simulink model "aocs"  (R2026a)
settings: Solver=VariableStepAuto  StopTime=500
values from neighbouring files (symbols this model uses):
  A = [0, 0, 0, 1, 0, 0 ... (first row only)    [aocs_controller.m]
  B = [zeros(3,3) ... (first row only)    [aocs_controller.m]
  C = eye(6, 6)    [aocs_controller.m]
  D = zeros(6, 3)    [aocs_controller.m]
  K = lqr(A,B,Q,R)    [aocs_controller.m]
settings Model: Creator=syane  LastModifiedBy=syane

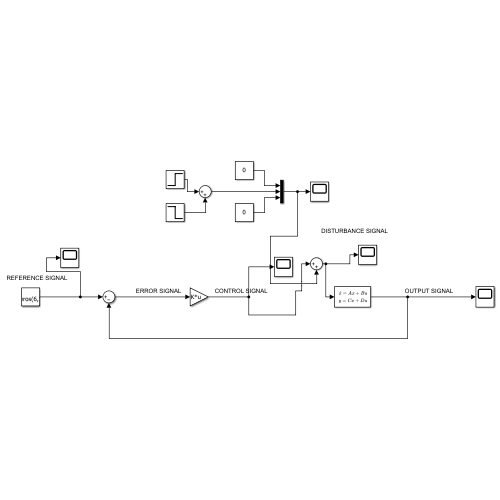
[thumbnail: Simulink's stored preview of the top-level diagram]
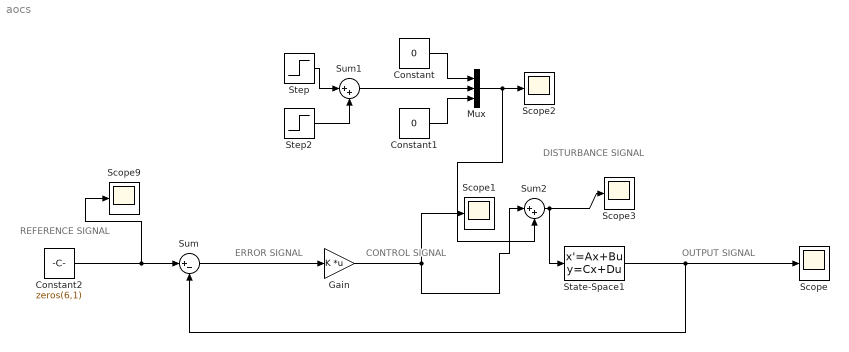
== system aocs ==
  note: DISTURBANCE SIGNAL
  note: CONTROL SIGNAL
  note: ERROR SIGNAL
  note: OUTPUT SIGNAL
  note: REFERENCE SIGNAL
  Constant : Constant  Value=0
  Constant1 : Constant  Value=0
  Constant2 : Constant  Value=zeros(6,1)
  Gain : Gain  Gain=K  Multiplication=Matrix(K*u)
  Mux : Mux  Inputs=3
  Scope{,1..3,9} (5 alike) : Scope
      Scope settings: ActiveDisplayYMinimum=-0.1683924744563659  ActiveDisplayYMaximum=1.0984465466181219
      Scope1 settings: ActiveDisplayYMinimum=-3.3931624331729169  ActiveDisplayYMaximum=0.60127720744566848
      Scope2 settings: ActiveDisplayYMinimum=-16.40625  ActiveDisplayYMaximum=101.18534482758621  DataLoggingVariableName=ScopeData2
      Scope3 settings: ActiveDisplayYMinimum=-15.867933277749938  ActiveDisplayYMaximum=112.87421480863888  DataLoggingVariableName=ScopeData3
      Scope9 settings: ActiveDisplayYMinimum=-1  ActiveDisplayYMaximum=1  DataLoggingVariableName=ScopeData9
  State-Space1 : StateSpace  A=A  B=B  C=C  D=D  InitialCondition=0
  Step : Step  FinalValue=100  SampleTime=0
  Step2 : Step  Time=2  FinalValue=-100  SampleTime=0
  Sum : Sum  Inputs=|+-
  Sum1 : Sum  Inputs=|++
  Sum2 : Sum  Inputs=|++
  wires:
  Constant1/1 -> Mux/3
  Constant/1 -> Mux/1
  Sum/1 -> Gain/1
  State-Space1/1 -> Sum/2, Scope/1
  Constant2/1 -> Scope9/1, Sum/1
  Mux/1 -> Sum2/2, Scope2/1
  Sum1/1 -> Mux/2
  Step2/1 -> Sum1/2
  Step/1 -> Sum1/1
  Sum2/1 -> State-Space1/1, Scope3/1
  Gain/1 -> Sum2/1, Scope1/1
